simulink model "IEEE5BusSystemModel_opt_UFLS"  (R2019b)
settings: Solver=ode4  StartTime=0.0  StopTime=300  MaxStep=1e-4  RelTol=1e-3
InitFcn:
  | startup_RTS
values from neighbouring files (symbols this model uses):
  C = b/(2*pi*60*Zn)    [startup_RTS.m]
  C0 = C/3    [startup_RTS.m]
  dPLS1 = 0    [startup_RTS.m]
  dPLS2 = 0    [startup_RTS.m]
  dPLS3 = 0    [startup_RTS.m]
  dQLS1 = 0    [startup_RTS.m]
  dQLS2 = 0    [startup_RTS.m]
  dQLS3 = 0    [startup_RTS.m]
  fn = 50    [startup_RTS.m]
  In = Sn/(sqrt(3)*Vn)    [startup_RTS.m]
  L = x*Zn/(2*pi*60)    [startup_RTS.m]
  L0 = 3*L    [startup_RTS.m]
  len = ceil(0.95*300000*T_prop)    [startup_RTS.m]
  PL1 = 300e6    (= 300000000)    [startup_RTS.m]
  PL2 = 300e6    (= 300000000)    [startup_RTS.m]
  PL3 = 300e6    (= 300000000)    [startup_RTS.m]
  QL1 = 30e6    (= 30000000)    [startup_RTS.m]
  QL2 = 30e6    (= 30000000)    [startup_RTS.m]
  QL3 = 30e6    (= 30000000)    [startup_RTS.m]
  R = r*Zn    [startup_RTS.m]
  R0 = 3*R    [startup_RTS.m]
  Sn = 1000e6    (= 1000000000)    [startup_RTS.m]
  t_cont = 100    [startup_RTS.m]
  Vn = 345e3    (= 345000)    [startup_RTS.m]
undefined symbols (not defined in the file or in its folder): D1, Delta
libraries: powerlib x42, dspswit3 x10, powerlib_meascontrol x3, dspstat3 x3, sps_avr x3, spsExcitationSystemModel x3
(part 3 of 7)

== system IEEE5BusSystemModel_opt_UFLS/Subsystem1/PMU_e-IpDFT_P-class1/Ia_est ==
  signal : Inport
  Hit : Inport  Port=2
  dT [s] : Inport  Port=3
  dF [Hz] : Inport  Port=4
  Synchrophasor estimation : Subsystem
  mSDFT : Subsystem
  Frequency : Outport  VectorParamsAs1DForOutWhenUnconnected=off
  Amplitude : Outport  Port=2  VectorParamsAs1DForOutWhenUnconnected=off
  Phase : Outport  Port=3  VectorParamsAs1DForOutWhenUnconnected=off
  wires:
  dF [Hz]/1 -> Synchrophasor estimation/3(dF [Hz])
  Synchrophasor estimation/1(Frequency) -> Frequency/1
  signal/1 -> mSDFT/1(signal)
  mSDFT/1(DFT) -> Synchrophasor estimation/1(DFT)
  Synchrophasor estimation/2(Amplitude) -> Amplitude/1
  Synchrophasor estimation/3(Phase) -> Phase/1
  Hit/1 -> mSDFT/2(Hit)
  dT [s]/1 -> Synchrophasor estimation/2(dT [s])

== system IEEE5BusSystemModel_opt_UFLS/Subsystem2/PMU_e-IpDFT_P-class/Ia_est ==
  signal : Inport
  Hit : Inport  Port=2
  dT [s] : Inport  Port=3
  dF [Hz] : Inport  Port=4
  Synchrophasor estimation : Subsystem
  mSDFT : Subsystem
  Frequency : Outport  VectorParamsAs1DForOutWhenUnconnected=off
  Amplitude : Outport  Port=2  VectorParamsAs1DForOutWhenUnconnected=off
  Phase : Outport  Port=3  VectorParamsAs1DForOutWhenUnconnected=off
  wires:
  dF [Hz]/1 -> Synchrophasor estimation/3(dF [Hz])
  Synchrophasor estimation/1(Frequency) -> Frequency/1
  signal/1 -> mSDFT/1(signal)
  mSDFT/1(DFT) -> Synchrophasor estimation/1(DFT)
  Synchrophasor estimation/2(Amplitude) -> Amplitude/1
  Synchrophasor estimation/3(Phase) -> Phase/1
  Hit/1 -> mSDFT/2(Hit)
  dT [s]/1 -> Synchrophasor estimation/2(dT [s])

== system IEEE5BusSystemModel_opt_UFLS/Subsystem2/PMU_e-IpDFT_P-class1/Ia_est ==
  signal : Inport
  Hit : Inport  Port=2
  dT [s] : Inport  Port=3
  dF [Hz] : Inport  Port=4
  Synchrophasor estimation : Subsystem
  mSDFT : Subsystem
  Frequency : Outport  VectorParamsAs1DForOutWhenUnconnected=off
  Amplitude : Outport  Port=2  VectorParamsAs1DForOutWhenUnconnected=off
  Phase : Outport  Port=3  VectorParamsAs1DForOutWhenUnconnected=off
  wires:
  dT [s]/1 -> Synchrophasor estimation/2(dT [s])
  Hit/1 -> mSDFT/2(Hit)
  Synchrophasor estimation/3(Phase) -> Phase/1
  Synchrophasor estimation/2(Amplitude) -> Amplitude/1
  mSDFT/1(DFT) -> Synchrophasor estimation/1(DFT)
  signal/1 -> mSDFT/1(signal)
  Synchrophasor estimation/1(Frequency) -> Frequency/1
  dF [Hz]/1 -> Synchrophasor estimation/3(dF [Hz])

== system IEEE5BusSystemModel_opt_UFLS/Subsystem3/PMU_e-IpDFT_P-class/Ia_est ==
  signal : Inport
  Hit : Inport  Port=2
  dT [s] : Inport  Port=3
  dF [Hz] : Inport  Port=4
  Synchrophasor estimation : Subsystem
  mSDFT : Subsystem
  Frequency : Outport  VectorParamsAs1DForOutWhenUnconnected=off
  Amplitude : Outport  Port=2  VectorParamsAs1DForOutWhenUnconnected=off
  Phase : Outport  Port=3  VectorParamsAs1DForOutWhenUnconnected=off
  wires:
  dT [s]/1 -> Synchrophasor estimation/2(dT [s])
  Hit/1 -> mSDFT/2(Hit)
  Synchrophasor estimation/3(Phase) -> Phase/1
  Synchrophasor estimation/2(Amplitude) -> Amplitude/1
  mSDFT/1(DFT) -> Synchrophasor estimation/1(DFT)
  signal/1 -> mSDFT/1(signal)
  Synchrophasor estimation/1(Frequency) -> Frequency/1
  dF [Hz]/1 -> Synchrophasor estimation/3(dF [Hz])

== system IEEE5BusSystemModel_opt_UFLS/Subsystem3/PMU_e-IpDFT_P-class1/Ia_est ==
  signal : Inport
  Hit : Inport  Port=2
  dT [s] : Inport  Port=3
  dF [Hz] : Inport  Port=4
  Synchrophasor estimation : Subsystem
  mSDFT : Subsystem
  Frequency : Outport  VectorParamsAs1DForOutWhenUnconnected=off
  Amplitude : Outport  Port=2  VectorParamsAs1DForOutWhenUnconnected=off
  Phase : Outport  Port=3  VectorParamsAs1DForOutWhenUnconnected=off
  wires:
  dF [Hz]/1 -> Synchrophasor estimation/3(dF [Hz])
  Synchrophasor estimation/1(Frequency) -> Frequency/1
  signal/1 -> mSDFT/1(signal)
  mSDFT/1(DFT) -> Synchrophasor estimation/1(DFT)
  Synchrophasor estimation/2(Amplitude) -> Amplitude/1
  Synchrophasor estimation/3(Phase) -> Phase/1
  Hit/1 -> mSDFT/2(Hit)
  dT [s]/1 -> Synchrophasor estimation/2(dT [s])

== system IEEE5BusSystemModel_opt_UFLS/Subsystem4/PMU_e-IpDFT_P-class/Ia_est ==
  signal : Inport
  Hit : Inport  Port=2
  dT [s] : Inport  Port=3
  dF [Hz] : Inport  Port=4
  Synchrophasor estimation : Subsystem
  mSDFT : Subsystem
  Frequency : Outport  VectorParamsAs1DForOutWhenUnconnected=off
  Amplitude : Outport  Port=2  VectorParamsAs1DForOutWhenUnconnected=off
  Phase : Outport  Port=3  VectorParamsAs1DForOutWhenUnconnected=off
  wires:
  dF [Hz]/1 -> Synchrophasor estimation/3(dF [Hz])
  Synchrophasor estimation/1(Frequency) -> Frequency/1
  signal/1 -> mSDFT/1(signal)
  mSDFT/1(DFT) -> Synchrophasor estimation/1(DFT)
  Synchrophasor estimation/2(Amplitude) -> Amplitude/1
  Synchrophasor estimation/3(Phase) -> Phase/1
  Hit/1 -> mSDFT/2(Hit)
  dT [s]/1 -> Synchrophasor estimation/2(dT [s])

== system IEEE5BusSystemModel_opt_UFLS/Subsystem4/PMU_e-IpDFT_P-class1/Ia_est ==
  signal : Inport
  Hit : Inport  Port=2
  dT [s] : Inport  Port=3
  dF [Hz] : Inport  Port=4
  Synchrophasor estimation : Subsystem
  mSDFT : Subsystem
  Frequency : Outport  VectorParamsAs1DForOutWhenUnconnected=off
  Amplitude : Outport  Port=2  VectorParamsAs1DForOutWhenUnconnected=off
  Phase : Outport  Port=3  VectorParamsAs1DForOutWhenUnconnected=off
  wires:
  dT [s]/1 -> Synchrophasor estimation/2(dT [s])
  Hit/1 -> mSDFT/2(Hit)
  Synchrophasor estimation/3(Phase) -> Phase/1
  Synchrophasor estimation/2(Amplitude) -> Amplitude/1
  mSDFT/1(DFT) -> Synchrophasor estimation/1(DFT)
  signal/1 -> mSDFT/1(signal)
  Synchrophasor estimation/1(Frequency) -> Frequency/1
  dF [Hz]/1 -> Synchrophasor estimation/3(dF [Hz])

== system IEEE5BusSystemModel_opt_UFLS/Subsystem5/PMU_e-IpDFT_P-class/Ia_est ==
  signal : Inport
  Hit : Inport  Port=2
  dT [s] : Inport  Port=3
  dF [Hz] : Inport  Port=4
  Synchrophasor estimation : Subsystem
  mSDFT : Subsystem
  Frequency : Outport  VectorParamsAs1DForOutWhenUnconnected=off
  Amplitude : Outport  Port=2  VectorParamsAs1DForOutWhenUnconnected=off
  Phase : Outport  Port=3  VectorParamsAs1DForOutWhenUnconnected=off
  wires:
  dF [Hz]/1 -> Synchrophasor estimation/3(dF [Hz])
  Synchrophasor estimation/1(Frequency) -> Frequency/1
  signal/1 -> mSDFT/1(signal)
  mSDFT/1(DFT) -> Synchrophasor estimation/1(DFT)
  Synchrophasor estimation/2(Amplitude) -> Amplitude/1
  Synchrophasor estimation/3(Phase) -> Phase/1
  Hit/1 -> mSDFT/2(Hit)
  dT [s]/1 -> Synchrophasor estimation/2(dT [s])

== system IEEE5BusSystemModel_opt_UFLS/Subsystem5/PMU_e-IpDFT_P-class1/Ia_est ==
  signal : Inport
  Hit : Inport  Port=2
  dT [s] : Inport  Port=3
  dF [Hz] : Inport  Port=4
  Synchrophasor estimation : Subsystem
  mSDFT : Subsystem
  Frequency : Outport  VectorParamsAs1DForOutWhenUnconnected=off
  Amplitude : Outport  Port=2  VectorParamsAs1DForOutWhenUnconnected=off
  Phase : Outport  Port=3  VectorParamsAs1DForOutWhenUnconnected=off
  wires:
  dT [s]/1 -> Synchrophasor estimation/2(dT [s])
  Hit/1 -> mSDFT/2(Hit)
  Synchrophasor estimation/3(Phase) -> Phase/1
  Synchrophasor estimation/2(Amplitude) -> Amplitude/1
  mSDFT/1(DFT) -> Synchrophasor estimation/1(DFT)
  signal/1 -> mSDFT/1(signal)
  Synchrophasor estimation/1(Frequency) -> Frequency/1
  dF [Hz]/1 -> Synchrophasor estimation/3(dF [Hz])

== system IEEE5BusSystemModel_opt_UFLS/Subsystem1/PMU_e-IpDFT_P-class/Ia_est/Synchrophasor estimation ==
  DFT : Inport
  dT [s] : Inport  Port=2
  dF [Hz] : Inport  Port=3
  Amplitude - 1 : Subsystem
  Amplitude - 2 : Subsystem
  Complex to Magnitude-Angle1 : ComplexToMagnitudeAngle
  Complex to Magnitude-Angle2 : ComplexToMagnitudeAngle
  Demux1 : Demux  Outputs=5
  Frequency - 2 : Subsystem
  Hanning(Kmax) : Subsystem
  Hanning(Kmax+1) : Subsystem
  Hanning(Kmax-1) : Subsystem
  Phase - 2 : Subsystem
  Terminator : Terminator
  Terminator1 : Terminator
  "delta - 1 " : Subsystem
  delta - 2 : Subsystem
  epsilon : Subsystem
  spectral leakage compensation : Subsystem
  Frequency : Outport  VectorParamsAs1DForOutWhenUnconnected=off
  Amplitude : Outport  Port=2  VectorParamsAs1DForOutWhenUnconnected=off
  Phase : Outport  Port=3  VectorParamsAs1DForOutWhenUnconnected=off
  wires:
  DFT/1 -> Demux1/1
  Frequency - 2/1(frequency) -> Phase - 2/3(freq), Frequency/1
  Amplitude - 2/1(amplitude) -> Amplitude/1
  Demux1/5 -> Hanning(Kmax+1)/3(Kmax+2)
  Demux1/1 -> Hanning(Kmax-1)/1(Kmax-2)
  Demux1/2 -> Hanning(Kmax)/1(Kmax-1), Hanning(Kmax-1)/2(Kmax-1)
  Demux1/3 -> Hanning(Kmax-1)/3(Kmax), Hanning(Kmax+1)/1(Kmax), Hanning(Kmax)/2(Kmax)
  Demux1/4 -> Hanning(Kmax+1)/2(Kmax+1), Hanning(Kmax)/3(Kmax+1)
  Hanning(Kmax+1)/1(Hanning out) -> epsilon/2(X (k max+1))
  Hanning(Kmax)/1(Hanning out) -> "delta - 1 "/1(X (k max)), Amplitude - 1/2((X k_max)), spectral leakage compensation/4(X (k max))
  epsilon/1(X (Kmax + epsilon)) -> "delta - 1 "/2(X (k max + epsilon)), spectral leakage compensation/3(X (k max + epsilon))
  epsilon/2(epsilon) -> spectral leakage compensation/5(epsilon), delta - 2/3(epsilon), "delta - 1 "/3(epsilon)
  "delta - 1 "/1(delta) -> spectral leakage compensation/2(delta), Amplitude - 1/1(delta)
  spectral leakage compensation/1(X(k max)) -> delta - 2/1(X (k max)), Complex to Magnitude-Angle2/1, Amplitude - 2/2((X k_max))
  spectral leakage compensation/2(X(k max+epsilon)) -> delta - 2/2(X (k max + epsilon))
  delta - 2/1(delta) -> Frequency - 2/1(delta), Phase - 2/2(delta), Amplitude - 2/1(delta)
  Phase - 2/1(phase) -> Phase/1
  Complex to Magnitude-Angle1/2 -> spectral leakage compensation/6(ph X(k-1))
  Complex to Magnitude-Angle1/1 -> Terminator/1
  Complex to Magnitude-Angle2/2 -> Phase - 2/1(X k_max phase)
  Complex to Magnitude-Angle2/1 -> Terminator1/1
  dT [s]/1 -> Phase - 2/4(dT [s])
  Amplitude - 1/1(amplitude) -> spectral leakage compensation/1(Amplitude)
  Hanning(Kmax-1)/1(Hanning out) -> Complex to Magnitude-Angle1/1, epsilon/1(X (k max -1))
  dF [Hz]/1 -> Frequency - 2/2(dF [Hz])

== system IEEE5BusSystemModel_opt_UFLS/Subsystem1/PMU_e-IpDFT_P-class/Ia_est/mSDFT ==
  signal : Inport
  Hit : Inport  Port=2
  Delay_M : Delay  DelayLength=M  SampleTime=Ts_p
  Kmax : Subsystem
  Kmax+1 : Subsystem
  Kmax+2 : Subsystem
  Kmax-1 : Subsystem
  Kmax-2 : Subsystem
  Mux : Mux  Inputs=5
  DFT : Outport  VectorParamsAs1DForOutWhenUnconnected=off
  wires:
  Mux/1 -> DFT/1
  Kmax+2/1(X(k)) -> Mux/5
  Kmax+1/1(X(k)) -> Mux/4
  Kmax/1(X(k)) -> Mux/3
  Kmax-1/1(X(k)) -> Mux/2
  Kmax-2/1(X(k)) -> Mux/1
  signal/1 -> Kmax-2/1(x(n)), Kmax-1/1(x(n)), Kmax+2/1(x(n)), Kmax+1/1(x(n)), Kmax/1(x(n)), Delay_M/1
  Delay_M/1 -> Kmax/2(x(n-M)), Kmax+1/2(x(n-M)), Kmax+2/2(x(n-M)), Kmax-1/2(x(n-M)), Kmax-2/2(x(n-M))
  Hit/1 -> Kmax-2/3(trigger), Kmax-1/3(trigger), Kmax/3(trigger), Kmax+1/3(trigger), Kmax+2/3(trigger)

== system IEEE5BusSystemModel_opt_UFLS/Subsystem1/PMU_e-IpDFT_P-class1/Ia_est/Synchrophasor estimation ==
  DFT : Inport
  dT [s] : Inport  Port=2
  dF [Hz] : Inport  Port=3
  Amplitude - 1 : Subsystem
  Amplitude - 2 : Subsystem
  Complex to Magnitude-Angle1 : ComplexToMagnitudeAngle
  Complex to Magnitude-Angle2 : ComplexToMagnitudeAngle
  Demux1 : Demux  Outputs=5
  Frequency - 2 : Subsystem
  Hanning(Kmax) : Subsystem
  Hanning(Kmax+1) : Subsystem
  Hanning(Kmax-1) : Subsystem
  Phase - 2 : Subsystem
  Terminator : Terminator
  Terminator1 : Terminator
  "delta - 1 " : Subsystem
  delta - 2 : Subsystem
  epsilon : Subsystem
  spectral leakage compensation : Subsystem
  Frequency : Outport  VectorParamsAs1DForOutWhenUnconnected=off
  Amplitude : Outport  Port=2  VectorParamsAs1DForOutWhenUnconnected=off
  Phase : Outport  Port=3  VectorParamsAs1DForOutWhenUnconnected=off
  wires:
  dF [Hz]/1 -> Frequency - 2/2(dF [Hz])
  Hanning(Kmax-1)/1(Hanning out) -> epsilon/1(X (k max -1)), Complex to Magnitude-Angle1/1
  Amplitude - 1/1(amplitude) -> spectral leakage compensation/1(Amplitude)
  dT [s]/1 -> Phase - 2/4(dT [s])
  Complex to Magnitude-Angle2/1 -> Terminator1/1
  Complex to Magnitude-Angle2/2 -> Phase - 2/1(X k_max phase)
  Complex to Magnitude-Angle1/1 -> Terminator/1
  Complex to Magnitude-Angle1/2 -> spectral leakage compensation/6(ph X(k-1))
  Phase - 2/1(phase) -> Phase/1
  delta - 2/1(delta) -> Amplitude - 2/1(delta), Phase - 2/2(delta), Frequency - 2/1(delta)
  spectral leakage compensation/2(X(k max+epsilon)) -> delta - 2/2(X (k max + epsilon))
  spectral leakage compensation/1(X(k max)) -> Amplitude - 2/2((X k_max)), Complex to Magnitude-Angle2/1, delta - 2/1(X (k max))
  "delta - 1 "/1(delta) -> Amplitude - 1/1(delta), spectral leakage compensation/2(delta)
  epsilon/2(epsilon) -> "delta - 1 "/3(epsilon), delta - 2/3(epsilon), spectral leakage compensation/5(epsilon)
  epsilon/1(X (Kmax + epsilon)) -> spectral leakage compensation/3(X (k max + epsilon)), "delta - 1 "/2(X (k max + epsilon))
  Hanning(Kmax)/1(Hanning out) -> spectral leakage compensation/4(X (k max)), Amplitude - 1/2((X k_max)), "delta - 1 "/1(X (k max))
  Hanning(Kmax+1)/1(Hanning out) -> epsilon/2(X (k max+1))
  Demux1/4 -> Hanning(Kmax)/3(Kmax+1), Hanning(Kmax+1)/2(Kmax+1)
  Demux1/3 -> Hanning(Kmax)/2(Kmax), Hanning(Kmax+1)/1(Kmax), Hanning(Kmax-1)/3(Kmax)
  Demux1/2 -> Hanning(Kmax-1)/2(Kmax-1), Hanning(Kmax)/1(Kmax-1)
  Demux1/1 -> Hanning(Kmax-1)/1(Kmax-2)
  Demux1/5 -> Hanning(Kmax+1)/3(Kmax+2)
  Amplitude - 2/1(amplitude) -> Amplitude/1
  Frequency - 2/1(frequency) -> Frequency/1, Phase - 2/3(freq)
  DFT/1 -> Demux1/1

== system IEEE5BusSystemModel_opt_UFLS/Subsystem1/PMU_e-IpDFT_P-class1/Ia_est/mSDFT ==
  signal : Inport
  Hit : Inport  Port=2
  Delay_M : Delay  DelayLength=M  SampleTime=Ts_p
  Kmax : Subsystem
  Kmax+1 : Subsystem
  Kmax+2 : Subsystem
  Kmax-1 : Subsystem
  Kmax-2 : Subsystem
  Mux : Mux  Inputs=5
  DFT : Outport  VectorParamsAs1DForOutWhenUnconnected=off
  wires:
  Hit/1 -> Kmax+2/3(trigger), Kmax+1/3(trigger), Kmax/3(trigger), Kmax-1/3(trigger), Kmax-2/3(trigger)
  Delay_M/1 -> Kmax-2/2(x(n-M)), Kmax-1/2(x(n-M)), Kmax+2/2(x(n-M)), Kmax+1/2(x(n-M)), Kmax/2(x(n-M))
  signal/1 -> Delay_M/1, Kmax/1(x(n)), Kmax+1/1(x(n)), Kmax+2/1(x(n)), Kmax-1/1(x(n)), Kmax-2/1(x(n))
  Kmax-2/1(X(k)) -> Mux/1
  Kmax-1/1(X(k)) -> Mux/2
  Kmax/1(X(k)) -> Mux/3
  Kmax+1/1(X(k)) -> Mux/4
  Kmax+2/1(X(k)) -> Mux/5
  Mux/1 -> DFT/1

== system IEEE5BusSystemModel_opt_UFLS/Subsystem2/PMU_e-IpDFT_P-class/Ia_est/Synchrophasor estimation ==
  DFT : Inport
  dT [s] : Inport  Port=2
  dF [Hz] : Inport  Port=3
  Amplitude - 1 : Subsystem
  Amplitude - 2 : Subsystem
  Complex to Magnitude-Angle1 : ComplexToMagnitudeAngle
  Complex to Magnitude-Angle2 : ComplexToMagnitudeAngle
  Demux1 : Demux  Outputs=5
  Frequency - 2 : Subsystem
  Hanning(Kmax) : Subsystem
  Hanning(Kmax+1) : Subsystem
  Hanning(Kmax-1) : Subsystem
  Phase - 2 : Subsystem
  Terminator : Terminator
  Terminator1 : Terminator
  "delta - 1 " : Subsystem
  delta - 2 : Subsystem
  epsilon : Subsystem
  spectral leakage compensation : Subsystem
  Frequency : Outport  VectorParamsAs1DForOutWhenUnconnected=off
  Amplitude : Outport  Port=2  VectorParamsAs1DForOutWhenUnconnected=off
  Phase : Outport  Port=3  VectorParamsAs1DForOutWhenUnconnected=off
  wires:
  dF [Hz]/1 -> Frequency - 2/2(dF [Hz])
  Hanning(Kmax-1)/1(Hanning out) -> epsilon/1(X (k max -1)), Complex to Magnitude-Angle1/1
  Amplitude - 1/1(amplitude) -> spectral leakage compensation/1(Amplitude)
  dT [s]/1 -> Phase - 2/4(dT [s])
  Complex to Magnitude-Angle2/1 -> Terminator1/1
  Complex to Magnitude-Angle2/2 -> Phase - 2/1(X k_max phase)
  Complex to Magnitude-Angle1/1 -> Terminator/1
  Complex to Magnitude-Angle1/2 -> spectral leakage compensation/6(ph X(k-1))
  Phase - 2/1(phase) -> Phase/1
  delta - 2/1(delta) -> Amplitude - 2/1(delta), Phase - 2/2(delta), Frequency - 2/1(delta)
  spectral leakage compensation/2(X(k max+epsilon)) -> delta - 2/2(X (k max + epsilon))
  spectral leakage compensation/1(X(k max)) -> Amplitude - 2/2((X k_max)), Complex to Magnitude-Angle2/1, delta - 2/1(X (k max))
  "delta - 1 "/1(delta) -> Amplitude - 1/1(delta), spectral leakage compensation/2(delta)
  epsilon/2(epsilon) -> "delta - 1 "/3(epsilon), delta - 2/3(epsilon), spectral leakage compensation/5(epsilon)
  epsilon/1(X (Kmax + epsilon)) -> spectral leakage compensation/3(X (k max + epsilon)), "delta - 1 "/2(X (k max + epsilon))
  Hanning(Kmax)/1(Hanning out) -> spectral leakage compensation/4(X (k max)), Amplitude - 1/2((X k_max)), "delta - 1 "/1(X (k max))
  Hanning(Kmax+1)/1(Hanning out) -> epsilon/2(X (k max+1))
  Demux1/4 -> Hanning(Kmax)/3(Kmax+1), Hanning(Kmax+1)/2(Kmax+1)
  Demux1/3 -> Hanning(Kmax)/2(Kmax), Hanning(Kmax+1)/1(Kmax), Hanning(Kmax-1)/3(Kmax)
  Demux1/2 -> Hanning(Kmax-1)/2(Kmax-1), Hanning(Kmax)/1(Kmax-1)
  Demux1/1 -> Hanning(Kmax-1)/1(Kmax-2)
  Demux1/5 -> Hanning(Kmax+1)/3(Kmax+2)
  Amplitude - 2/1(amplitude) -> Amplitude/1
  Frequency - 2/1(frequency) -> Frequency/1, Phase - 2/3(freq)
  DFT/1 -> Demux1/1

== system IEEE5BusSystemModel_opt_UFLS/Subsystem2/PMU_e-IpDFT_P-class/Ia_est/mSDFT ==
  signal : Inport
  Hit : Inport  Port=2
  Delay_M : Delay  DelayLength=M  SampleTime=Ts_p
  Kmax : Subsystem
  Kmax+1 : Subsystem
  Kmax+2 : Subsystem
  Kmax-1 : Subsystem
  Kmax-2 : Subsystem
  Mux : Mux  Inputs=5
  DFT : Outport  VectorParamsAs1DForOutWhenUnconnected=off
  wires:
  Hit/1 -> Kmax+2/3(trigger), Kmax+1/3(trigger), Kmax/3(trigger), Kmax-1/3(trigger), Kmax-2/3(trigger)
  Delay_M/1 -> Kmax-2/2(x(n-M)), Kmax-1/2(x(n-M)), Kmax+2/2(x(n-M)), Kmax+1/2(x(n-M)), Kmax/2(x(n-M))
  signal/1 -> Delay_M/1, Kmax/1(x(n)), Kmax+1/1(x(n)), Kmax+2/1(x(n)), Kmax-1/1(x(n)), Kmax-2/1(x(n))
  Kmax-2/1(X(k)) -> Mux/1
  Kmax-1/1(X(k)) -> Mux/2
  Kmax/1(X(k)) -> Mux/3
  Kmax+1/1(X(k)) -> Mux/4
  Kmax+2/1(X(k)) -> Mux/5
  Mux/1 -> DFT/1

== system IEEE5BusSystemModel_opt_UFLS/Subsystem2/PMU_e-IpDFT_P-class1/Ia_est/Synchrophasor estimation ==
  DFT : Inport
  dT [s] : Inport  Port=2
  dF [Hz] : Inport  Port=3
  Amplitude - 1 : Subsystem
  Amplitude - 2 : Subsystem
  Complex to Magnitude-Angle1 : ComplexToMagnitudeAngle
  Complex to Magnitude-Angle2 : ComplexToMagnitudeAngle
  Demux1 : Demux  Outputs=5
  Frequency - 2 : Subsystem
  Hanning(Kmax) : Subsystem
  Hanning(Kmax+1) : Subsystem
  Hanning(Kmax-1) : Subsystem
  Phase - 2 : Subsystem
  Terminator : Terminator
  Terminator1 : Terminator
  "delta - 1 " : Subsystem
  delta - 2 : Subsystem
  epsilon : Subsystem
  spectral leakage compensation : Subsystem
  Frequency : Outport  VectorParamsAs1DForOutWhenUnconnected=off
  Amplitude : Outport  Port=2  VectorParamsAs1DForOutWhenUnconnected=off
  Phase : Outport  Port=3  VectorParamsAs1DForOutWhenUnconnected=off
  wires:
  DFT/1 -> Demux1/1
  Frequency - 2/1(frequency) -> Phase - 2/3(freq), Frequency/1
  Amplitude - 2/1(amplitude) -> Amplitude/1
  Demux1/5 -> Hanning(Kmax+1)/3(Kmax+2)
  Demux1/1 -> Hanning(Kmax-1)/1(Kmax-2)
  Demux1/2 -> Hanning(Kmax)/1(Kmax-1), Hanning(Kmax-1)/2(Kmax-1)
  Demux1/3 -> Hanning(Kmax-1)/3(Kmax), Hanning(Kmax+1)/1(Kmax), Hanning(Kmax)/2(Kmax)
  Demux1/4 -> Hanning(Kmax+1)/2(Kmax+1), Hanning(Kmax)/3(Kmax+1)
  Hanning(Kmax+1)/1(Hanning out) -> epsilon/2(X (k max+1))
  Hanning(Kmax)/1(Hanning out) -> "delta - 1 "/1(X (k max)), Amplitude - 1/2((X k_max)), spectral leakage compensation/4(X (k max))
  epsilon/1(X (Kmax + epsilon)) -> "delta - 1 "/2(X (k max + epsilon)), spectral leakage compensation/3(X (k max + epsilon))
  epsilon/2(epsilon) -> spectral leakage compensation/5(epsilon), delta - 2/3(epsilon), "delta - 1 "/3(epsilon)
  "delta - 1 "/1(delta) -> spectral leakage compensation/2(delta), Amplitude - 1/1(delta)
  spectral leakage compensation/1(X(k max)) -> delta - 2/1(X (k max)), Complex to Magnitude-Angle2/1, Amplitude - 2/2((X k_max))
  spectral leakage compensation/2(X(k max+epsilon)) -> delta - 2/2(X (k max + epsilon))
  delta - 2/1(delta) -> Frequency - 2/1(delta), Phase - 2/2(delta), Amplitude - 2/1(delta)
  Phase - 2/1(phase) -> Phase/1
  Complex to Magnitude-Angle1/2 -> spectral leakage compensation/6(ph X(k-1))
  Complex to Magnitude-Angle1/1 -> Terminator/1
  Complex to Magnitude-Angle2/2 -> Phase - 2/1(X k_max phase)
  Complex to Magnitude-Angle2/1 -> Terminator1/1
  dT [s]/1 -> Phase - 2/4(dT [s])
  Amplitude - 1/1(amplitude) -> spectral leakage compensation/1(Amplitude)
  Hanning(Kmax-1)/1(Hanning out) -> Complex to Magnitude-Angle1/1, epsilon/1(X (k max -1))
  dF [Hz]/1 -> Frequency - 2/2(dF [Hz])

== system IEEE5BusSystemModel_opt_UFLS/Subsystem2/PMU_e-IpDFT_P-class1/Ia_est/mSDFT ==
  signal : Inport
  Hit : Inport  Port=2
  Delay_M : Delay  DelayLength=M  SampleTime=Ts_p
  Kmax : Subsystem
  Kmax+1 : Subsystem
  Kmax+2 : Subsystem
  Kmax-1 : Subsystem
  Kmax-2 : Subsystem
  Mux : Mux  Inputs=5
  DFT : Outport  VectorParamsAs1DForOutWhenUnconnected=off
  wires:
  Mux/1 -> DFT/1
  Kmax+2/1(X(k)) -> Mux/5
  Kmax+1/1(X(k)) -> Mux/4
  Kmax/1(X(k)) -> Mux/3
  Kmax-1/1(X(k)) -> Mux/2
  Kmax-2/1(X(k)) -> Mux/1
  signal/1 -> Kmax-2/1(x(n)), Kmax-1/1(x(n)), Kmax+2/1(x(n)), Kmax+1/1(x(n)), Kmax/1(x(n)), Delay_M/1
  Delay_M/1 -> Kmax/2(x(n-M)), Kmax+1/2(x(n-M)), Kmax+2/2(x(n-M)), Kmax-1/2(x(n-M)), Kmax-2/2(x(n-M))
  Hit/1 -> Kmax-2/3(trigger), Kmax-1/3(trigger), Kmax/3(trigger), Kmax+1/3(trigger), Kmax+2/3(trigger)

== system IEEE5BusSystemModel_opt_UFLS/Subsystem3/PMU_e-IpDFT_P-class/Ia_est/Synchrophasor estimation ==
  DFT : Inport
  dT [s] : Inport  Port=2
  dF [Hz] : Inport  Port=3
  Amplitude - 1 : Subsystem
  Amplitude - 2 : Subsystem
  Complex to Magnitude-Angle1 : ComplexToMagnitudeAngle
  Complex to Magnitude-Angle2 : ComplexToMagnitudeAngle
  Demux1 : Demux  Outputs=5
  Frequency - 2 : Subsystem
  Hanning(Kmax) : Subsystem
  Hanning(Kmax+1) : Subsystem
  Hanning(Kmax-1) : Subsystem
  Phase - 2 : Subsystem
  Terminator : Terminator
  Terminator1 : Terminator
  "delta - 1 " : Subsystem
  delta - 2 : Subsystem
  epsilon : Subsystem
  spectral leakage compensation : Subsystem
  Frequency : Outport  VectorParamsAs1DForOutWhenUnconnected=off
  Amplitude : Outport  Port=2  VectorParamsAs1DForOutWhenUnconnected=off
  Phase : Outport  Port=3  VectorParamsAs1DForOutWhenUnconnected=off
  wires:
  DFT/1 -> Demux1/1
  Frequency - 2/1(frequency) -> Phase - 2/3(freq), Frequency/1
  Amplitude - 2/1(amplitude) -> Amplitude/1
  Demux1/5 -> Hanning(Kmax+1)/3(Kmax+2)
  Demux1/1 -> Hanning(Kmax-1)/1(Kmax-2)
  Demux1/2 -> Hanning(Kmax)/1(Kmax-1), Hanning(Kmax-1)/2(Kmax-1)
  Demux1/3 -> Hanning(Kmax-1)/3(Kmax), Hanning(Kmax+1)/1(Kmax), Hanning(Kmax)/2(Kmax)
  Demux1/4 -> Hanning(Kmax+1)/2(Kmax+1), Hanning(Kmax)/3(Kmax+1)
  Hanning(Kmax+1)/1(Hanning out) -> epsilon/2(X (k max+1))
  Hanning(Kmax)/1(Hanning out) -> "delta - 1 "/1(X (k max)), Amplitude - 1/2((X k_max)), spectral leakage compensation/4(X (k max))
  epsilon/1(X (Kmax + epsilon)) -> "delta - 1 "/2(X (k max + epsilon)), spectral leakage compensation/3(X (k max + epsilon))
  epsilon/2(epsilon) -> spectral leakage compensation/5(epsilon), delta - 2/3(epsilon), "delta - 1 "/3(epsilon)
  "delta - 1 "/1(delta) -> spectral leakage compensation/2(delta), Amplitude - 1/1(delta)
  spectral leakage compensation/1(X(k max)) -> delta - 2/1(X (k max)), Complex to Magnitude-Angle2/1, Amplitude - 2/2((X k_max))
  spectral leakage compensation/2(X(k max+epsilon)) -> delta - 2/2(X (k max + epsilon))
  delta - 2/1(delta) -> Frequency - 2/1(delta), Phase - 2/2(delta), Amplitude - 2/1(delta)
  Phase - 2/1(phase) -> Phase/1
  Complex to Magnitude-Angle1/2 -> spectral leakage compensation/6(ph X(k-1))
  Complex to Magnitude-Angle1/1 -> Terminator/1
  Complex to Magnitude-Angle2/2 -> Phase - 2/1(X k_max phase)
  Complex to Magnitude-Angle2/1 -> Terminator1/1
  dT [s]/1 -> Phase - 2/4(dT [s])
  Amplitude - 1/1(amplitude) -> spectral leakage compensation/1(Amplitude)
  Hanning(Kmax-1)/1(Hanning out) -> Complex to Magnitude-Angle1/1, epsilon/1(X (k max -1))
  dF [Hz]/1 -> Frequency - 2/2(dF [Hz])

== system IEEE5BusSystemModel_opt_UFLS/Subsystem3/PMU_e-IpDFT_P-class/Ia_est/mSDFT ==
  signal : Inport
  Hit : Inport  Port=2
  Delay_M : Delay  DelayLength=M  SampleTime=Ts_p
  Kmax : Subsystem
  Kmax+1 : Subsystem
  Kmax+2 : Subsystem
  Kmax-1 : Subsystem
  Kmax-2 : Subsystem
  Mux : Mux  Inputs=5
  DFT : Outport  VectorParamsAs1DForOutWhenUnconnected=off
  wires:
  Mux/1 -> DFT/1
  Kmax+2/1(X(k)) -> Mux/5
  Kmax+1/1(X(k)) -> Mux/4
  Kmax/1(X(k)) -> Mux/3
  Kmax-1/1(X(k)) -> Mux/2
  Kmax-2/1(X(k)) -> Mux/1
  signal/1 -> Kmax-2/1(x(n)), Kmax-1/1(x(n)), Kmax+2/1(x(n)), Kmax+1/1(x(n)), Kmax/1(x(n)), Delay_M/1
  Delay_M/1 -> Kmax/2(x(n-M)), Kmax+1/2(x(n-M)), Kmax+2/2(x(n-M)), Kmax-1/2(x(n-M)), Kmax-2/2(x(n-M))
  Hit/1 -> Kmax-2/3(trigger), Kmax-1/3(trigger), Kmax/3(trigger), Kmax+1/3(trigger), Kmax+2/3(trigger)

== system IEEE5BusSystemModel_opt_UFLS/Subsystem3/PMU_e-IpDFT_P-class1/Ia_est/Synchrophasor estimation ==
  DFT : Inport
  dT [s] : Inport  Port=2
  dF [Hz] : Inport  Port=3
  Amplitude - 1 : Subsystem
  Amplitude - 2 : Subsystem
  Complex to Magnitude-Angle1 : ComplexToMagnitudeAngle
  Complex to Magnitude-Angle2 : ComplexToMagnitudeAngle
  Demux1 : Demux  Outputs=5
  Frequency - 2 : Subsystem
  Hanning(Kmax) : Subsystem
  Hanning(Kmax+1) : Subsystem
  Hanning(Kmax-1) : Subsystem
  Phase - 2 : Subsystem
  Terminator : Terminator
  Terminator1 : Terminator
  "delta - 1 " : Subsystem
  delta - 2 : Subsystem
  epsilon : Subsystem
  spectral leakage compensation : Subsystem
  Frequency : Outport  VectorParamsAs1DForOutWhenUnconnected=off
  Amplitude : Outport  Port=2  VectorParamsAs1DForOutWhenUnconnected=off
  Phase : Outport  Port=3  VectorParamsAs1DForOutWhenUnconnected=off
  wires:
  dF [Hz]/1 -> Frequency - 2/2(dF [Hz])
  Hanning(Kmax-1)/1(Hanning out) -> epsilon/1(X (k max -1)), Complex to Magnitude-Angle1/1
  Amplitude - 1/1(amplitude) -> spectral leakage compensation/1(Amplitude)
  dT [s]/1 -> Phase - 2/4(dT [s])
  Complex to Magnitude-Angle2/1 -> Terminator1/1
  Complex to Magnitude-Angle2/2 -> Phase - 2/1(X k_max phase)
  Complex to Magnitude-Angle1/1 -> Terminator/1
  Complex to Magnitude-Angle1/2 -> spectral leakage compensation/6(ph X(k-1))
  Phase - 2/1(phase) -> Phase/1
  delta - 2/1(delta) -> Amplitude - 2/1(delta), Phase - 2/2(delta), Frequency - 2/1(delta)
  spectral leakage compensation/2(X(k max+epsilon)) -> delta - 2/2(X (k max + epsilon))
  spectral leakage compensation/1(X(k max)) -> Amplitude - 2/2((X k_max)), Complex to Magnitude-Angle2/1, delta - 2/1(X (k max))
  "delta - 1 "/1(delta) -> Amplitude - 1/1(delta), spectral leakage compensation/2(delta)
  epsilon/2(epsilon) -> "delta - 1 "/3(epsilon), delta - 2/3(epsilon), spectral leakage compensation/5(epsilon)
  epsilon/1(X (Kmax + epsilon)) -> spectral leakage compensation/3(X (k max + epsilon)), "delta - 1 "/2(X (k max + epsilon))
  Hanning(Kmax)/1(Hanning out) -> spectral leakage compensation/4(X (k max)), Amplitude - 1/2((X k_max)), "delta - 1 "/1(X (k max))
  Hanning(Kmax+1)/1(Hanning out) -> epsilon/2(X (k max+1))
  Demux1/4 -> Hanning(Kmax)/3(Kmax+1), Hanning(Kmax+1)/2(Kmax+1)
  Demux1/3 -> Hanning(Kmax)/2(Kmax), Hanning(Kmax+1)/1(Kmax), Hanning(Kmax-1)/3(Kmax)
  Demux1/2 -> Hanning(Kmax-1)/2(Kmax-1), Hanning(Kmax)/1(Kmax-1)
  Demux1/1 -> Hanning(Kmax-1)/1(Kmax-2)
  Demux1/5 -> Hanning(Kmax+1)/3(Kmax+2)
  Amplitude - 2/1(amplitude) -> Amplitude/1
  Frequency - 2/1(frequency) -> Frequency/1, Phase - 2/3(freq)
  DFT/1 -> Demux1/1

== system IEEE5BusSystemModel_opt_UFLS/Subsystem3/PMU_e-IpDFT_P-class1/Ia_est/mSDFT ==
  signal : Inport
  Hit : Inport  Port=2
  Delay_M : Delay  DelayLength=M  SampleTime=Ts_p
  Kmax : Subsystem
  Kmax+1 : Subsystem
  Kmax+2 : Subsystem
  Kmax-1 : Subsystem
  Kmax-2 : Subsystem
  Mux : Mux  Inputs=5
  DFT : Outport  VectorParamsAs1DForOutWhenUnconnected=off
  wires:
  Hit/1 -> Kmax+2/3(trigger), Kmax+1/3(trigger), Kmax/3(trigger), Kmax-1/3(trigger), Kmax-2/3(trigger)
  Delay_M/1 -> Kmax-2/2(x(n-M)), Kmax-1/2(x(n-M)), Kmax+2/2(x(n-M)), Kmax+1/2(x(n-M)), Kmax/2(x(n-M))
  signal/1 -> Delay_M/1, Kmax/1(x(n)), Kmax+1/1(x(n)), Kmax+2/1(x(n)), Kmax-1/1(x(n)), Kmax-2/1(x(n))
  Kmax-2/1(X(k)) -> Mux/1
  Kmax-1/1(X(k)) -> Mux/2
  Kmax/1(X(k)) -> Mux/3
  Kmax+1/1(X(k)) -> Mux/4
  Kmax+2/1(X(k)) -> Mux/5
  Mux/1 -> DFT/1

== system IEEE5BusSystemModel_opt_UFLS/Subsystem4/PMU_e-IpDFT_P-class/Ia_est/Synchrophasor estimation ==
  DFT : Inport
  dT [s] : Inport  Port=2
  dF [Hz] : Inport  Port=3
  Amplitude - 1 : Subsystem
  Amplitude - 2 : Subsystem
  Complex to Magnitude-Angle1 : ComplexToMagnitudeAngle
  Complex to Magnitude-Angle2 : ComplexToMagnitudeAngle
  Demux1 : Demux  Outputs=5
  Frequency - 2 : Subsystem
  Hanning(Kmax) : Subsystem
  Hanning(Kmax+1) : Subsystem
  Hanning(Kmax-1) : Subsystem
  Phase - 2 : Subsystem
  Terminator : Terminator
  Terminator1 : Terminator
  "delta - 1 " : Subsystem
  delta - 2 : Subsystem
  epsilon : Subsystem
  spectral leakage compensation : Subsystem
  Frequency : Outport  VectorParamsAs1DForOutWhenUnconnected=off
  Amplitude : Outport  Port=2  VectorParamsAs1DForOutWhenUnconnected=off
  Phase : Outport  Port=3  VectorParamsAs1DForOutWhenUnconnected=off
  wires:
  dF [Hz]/1 -> Frequency - 2/2(dF [Hz])
  Hanning(Kmax-1)/1(Hanning out) -> epsilon/1(X (k max -1)), Complex to Magnitude-Angle1/1
  Amplitude - 1/1(amplitude) -> spectral leakage compensation/1(Amplitude)
  dT [s]/1 -> Phase - 2/4(dT [s])
  Complex to Magnitude-Angle2/1 -> Terminator1/1
  Complex to Magnitude-Angle2/2 -> Phase - 2/1(X k_max phase)
  Complex to Magnitude-Angle1/1 -> Terminator/1
  Complex to Magnitude-Angle1/2 -> spectral leakage compensation/6(ph X(k-1))
  Phase - 2/1(phase) -> Phase/1
  delta - 2/1(delta) -> Amplitude - 2/1(delta), Phase - 2/2(delta), Frequency - 2/1(delta)
  spectral leakage compensation/2(X(k max+epsilon)) -> delta - 2/2(X (k max + epsilon))
  spectral leakage compensation/1(X(k max)) -> Amplitude - 2/2((X k_max)), Complex to Magnitude-Angle2/1, delta - 2/1(X (k max))
  "delta - 1 "/1(delta) -> Amplitude - 1/1(delta), spectral leakage compensation/2(delta)
  epsilon/2(epsilon) -> "delta - 1 "/3(epsilon), delta - 2/3(epsilon), spectral leakage compensation/5(epsilon)
  epsilon/1(X (Kmax + epsilon)) -> spectral leakage compensation/3(X (k max + epsilon)), "delta - 1 "/2(X (k max + epsilon))
  Hanning(Kmax)/1(Hanning out) -> spectral leakage compensation/4(X (k max)), Amplitude - 1/2((X k_max)), "delta - 1 "/1(X (k max))
  Hanning(Kmax+1)/1(Hanning out) -> epsilon/2(X (k max+1))
  Demux1/4 -> Hanning(Kmax)/3(Kmax+1), Hanning(Kmax+1)/2(Kmax+1)
  Demux1/3 -> Hanning(Kmax)/2(Kmax), Hanning(Kmax+1)/1(Kmax), Hanning(Kmax-1)/3(Kmax)
  Demux1/2 -> Hanning(Kmax-1)/2(Kmax-1), Hanning(Kmax)/1(Kmax-1)
  Demux1/1 -> Hanning(Kmax-1)/1(Kmax-2)
  Demux1/5 -> Hanning(Kmax+1)/3(Kmax+2)
  Amplitude - 2/1(amplitude) -> Amplitude/1
  Frequency - 2/1(frequency) -> Frequency/1, Phase - 2/3(freq)
  DFT/1 -> Demux1/1

== system IEEE5BusSystemModel_opt_UFLS/Subsystem4/PMU_e-IpDFT_P-class/Ia_est/mSDFT ==
  signal : Inport
  Hit : Inport  Port=2
  Delay_M : Delay  DelayLength=M  SampleTime=Ts_p
  Kmax : Subsystem
  Kmax+1 : Subsystem
  Kmax+2 : Subsystem
  Kmax-1 : Subsystem
  Kmax-2 : Subsystem
  Mux : Mux  Inputs=5
  DFT : Outport  VectorParamsAs1DForOutWhenUnconnected=off
  wires:
  Hit/1 -> Kmax+2/3(trigger), Kmax+1/3(trigger), Kmax/3(trigger), Kmax-1/3(trigger), Kmax-2/3(trigger)
  Delay_M/1 -> Kmax-2/2(x(n-M)), Kmax-1/2(x(n-M)), Kmax+2/2(x(n-M)), Kmax+1/2(x(n-M)), Kmax/2(x(n-M))
  signal/1 -> Delay_M/1, Kmax/1(x(n)), Kmax+1/1(x(n)), Kmax+2/1(x(n)), Kmax-1/1(x(n)), Kmax-2/1(x(n))
  Kmax-2/1(X(k)) -> Mux/1
  Kmax-1/1(X(k)) -> Mux/2
  Kmax/1(X(k)) -> Mux/3
  Kmax+1/1(X(k)) -> Mux/4
  Kmax+2/1(X(k)) -> Mux/5
  Mux/1 -> DFT/1

== system IEEE5BusSystemModel_opt_UFLS/Subsystem4/PMU_e-IpDFT_P-class1/Ia_est/Synchrophasor estimation ==
  DFT : Inport
  dT [s] : Inport  Port=2
  dF [Hz] : Inport  Port=3
  Amplitude - 1 : Subsystem
  Amplitude - 2 : Subsystem
  Complex to Magnitude-Angle1 : ComplexToMagnitudeAngle
  Complex to Magnitude-Angle2 : ComplexToMagnitudeAngle
  Demux1 : Demux  Outputs=5
  Frequency - 2 : Subsystem
  Hanning(Kmax) : Subsystem
  Hanning(Kmax+1) : Subsystem
  Hanning(Kmax-1) : Subsystem
  Phase - 2 : Subsystem
  Terminator : Terminator
  Terminator1 : Terminator
  "delta - 1 " : Subsystem
  delta - 2 : Subsystem
  epsilon : Subsystem
  spectral leakage compensation : Subsystem
  Frequency : Outport  VectorParamsAs1DForOutWhenUnconnected=off
  Amplitude : Outport  Port=2  VectorParamsAs1DForOutWhenUnconnected=off
  Phase : Outport  Port=3  VectorParamsAs1DForOutWhenUnconnected=off
  wires:
  DFT/1 -> Demux1/1
  Frequency - 2/1(frequency) -> Phase - 2/3(freq), Frequency/1
  Amplitude - 2/1(amplitude) -> Amplitude/1
  Demux1/5 -> Hanning(Kmax+1)/3(Kmax+2)
  Demux1/1 -> Hanning(Kmax-1)/1(Kmax-2)
  Demux1/2 -> Hanning(Kmax)/1(Kmax-1), Hanning(Kmax-1)/2(Kmax-1)
  Demux1/3 -> Hanning(Kmax-1)/3(Kmax), Hanning(Kmax+1)/1(Kmax), Hanning(Kmax)/2(Kmax)
  Demux1/4 -> Hanning(Kmax+1)/2(Kmax+1), Hanning(Kmax)/3(Kmax+1)
  Hanning(Kmax+1)/1(Hanning out) -> epsilon/2(X (k max+1))
  Hanning(Kmax)/1(Hanning out) -> "delta - 1 "/1(X (k max)), Amplitude - 1/2((X k_max)), spectral leakage compensation/4(X (k max))
  epsilon/1(X (Kmax + epsilon)) -> "delta - 1 "/2(X (k max + epsilon)), spectral leakage compensation/3(X (k max + epsilon))
  epsilon/2(epsilon) -> spectral leakage compensation/5(epsilon), delta - 2/3(epsilon), "delta - 1 "/3(epsilon)
  "delta - 1 "/1(delta) -> spectral leakage compensation/2(delta), Amplitude - 1/1(delta)
  spectral leakage compensation/1(X(k max)) -> delta - 2/1(X (k max)), Complex to Magnitude-Angle2/1, Amplitude - 2/2((X k_max))
  spectral leakage compensation/2(X(k max+epsilon)) -> delta - 2/2(X (k max + epsilon))
  delta - 2/1(delta) -> Frequency - 2/1(delta), Phase - 2/2(delta), Amplitude - 2/1(delta)
  Phase - 2/1(phase) -> Phase/1
  Complex to Magnitude-Angle1/2 -> spectral leakage compensation/6(ph X(k-1))
  Complex to Magnitude-Angle1/1 -> Terminator/1
  Complex to Magnitude-Angle2/2 -> Phase - 2/1(X k_max phase)
  Complex to Magnitude-Angle2/1 -> Terminator1/1
  dT [s]/1 -> Phase - 2/4(dT [s])
  Amplitude - 1/1(amplitude) -> spectral leakage compensation/1(Amplitude)
  Hanning(Kmax-1)/1(Hanning out) -> Complex to Magnitude-Angle1/1, epsilon/1(X (k max -1))
  dF [Hz]/1 -> Frequency - 2/2(dF [Hz])

== system IEEE5BusSystemModel_opt_UFLS/Subsystem4/PMU_e-IpDFT_P-class1/Ia_est/mSDFT ==
  signal : Inport
  Hit : Inport  Port=2
  Delay_M : Delay  DelayLength=M  SampleTime=Ts_p
  Kmax : Subsystem
  Kmax+1 : Subsystem
  Kmax+2 : Subsystem
  Kmax-1 : Subsystem
  Kmax-2 : Subsystem
  Mux : Mux  Inputs=5
  DFT : Outport  VectorParamsAs1DForOutWhenUnconnected=off
  wires:
  Mux/1 -> DFT/1
  Kmax+2/1(X(k)) -> Mux/5
  Kmax+1/1(X(k)) -> Mux/4
  Kmax/1(X(k)) -> Mux/3
  Kmax-1/1(X(k)) -> Mux/2
  Kmax-2/1(X(k)) -> Mux/1
  signal/1 -> Kmax-2/1(x(n)), Kmax-1/1(x(n)), Kmax+2/1(x(n)), Kmax+1/1(x(n)), Kmax/1(x(n)), Delay_M/1
  Delay_M/1 -> Kmax/2(x(n-M)), Kmax+1/2(x(n-M)), Kmax+2/2(x(n-M)), Kmax-1/2(x(n-M)), Kmax-2/2(x(n-M))
  Hit/1 -> Kmax-2/3(trigger), Kmax-1/3(trigger), Kmax/3(trigger), Kmax+1/3(trigger), Kmax+2/3(trigger)

== system IEEE5BusSystemModel_opt_UFLS/Subsystem5/PMU_e-IpDFT_P-class/Ia_est/Synchrophasor estimation ==
  DFT : Inport
  dT [s] : Inport  Port=2
  dF [Hz] : Inport  Port=3
  Amplitude - 1 : Subsystem
  Amplitude - 2 : Subsystem
  Complex to Magnitude-Angle1 : ComplexToMagnitudeAngle
  Complex to Magnitude-Angle2 : ComplexToMagnitudeAngle
  Demux1 : Demux  Outputs=5
  Frequency - 2 : Subsystem
  Hanning(Kmax) : Subsystem
  Hanning(Kmax+1) : Subsystem
  Hanning(Kmax-1) : Subsystem
  Phase - 2 : Subsystem
  Terminator : Terminator
  Terminator1 : Terminator
  "delta - 1 " : Subsystem
  delta - 2 : Subsystem
  epsilon : Subsystem
  spectral leakage compensation : Subsystem
  Frequency : Outport  VectorParamsAs1DForOutWhenUnconnected=off
  Amplitude : Outport  Port=2  VectorParamsAs1DForOutWhenUnconnected=off
  Phase : Outport  Port=3  VectorParamsAs1DForOutWhenUnconnected=off
  wires:
  dF [Hz]/1 -> Frequency - 2/2(dF [Hz])
  Hanning(Kmax-1)/1(Hanning out) -> epsilon/1(X (k max -1)), Complex to Magnitude-Angle1/1
  Amplitude - 1/1(amplitude) -> spectral leakage compensation/1(Amplitude)
  dT [s]/1 -> Phase - 2/4(dT [s])
  Complex to Magnitude-Angle2/1 -> Terminator1/1
  Complex to Magnitude-Angle2/2 -> Phase - 2/1(X k_max phase)
  Complex to Magnitude-Angle1/1 -> Terminator/1
  Complex to Magnitude-Angle1/2 -> spectral leakage compensation/6(ph X(k-1))
  Phase - 2/1(phase) -> Phase/1
  delta - 2/1(delta) -> Amplitude - 2/1(delta), Phase - 2/2(delta), Frequency - 2/1(delta)
  spectral leakage compensation/2(X(k max+epsilon)) -> delta - 2/2(X (k max + epsilon))
  spectral leakage compensation/1(X(k max)) -> Amplitude - 2/2((X k_max)), Complex to Magnitude-Angle2/1, delta - 2/1(X (k max))
  "delta - 1 "/1(delta) -> Amplitude - 1/1(delta), spectral leakage compensation/2(delta)
  epsilon/2(epsilon) -> "delta - 1 "/3(epsilon), delta - 2/3(epsilon), spectral leakage compensation/5(epsilon)
  epsilon/1(X (Kmax + epsilon)) -> spectral leakage compensation/3(X (k max + epsilon)), "delta - 1 "/2(X (k max + epsilon))
  Hanning(Kmax)/1(Hanning out) -> spectral leakage compensation/4(X (k max)), Amplitude - 1/2((X k_max)), "delta - 1 "/1(X (k max))
  Hanning(Kmax+1)/1(Hanning out) -> epsilon/2(X (k max+1))
  Demux1/4 -> Hanning(Kmax)/3(Kmax+1), Hanning(Kmax+1)/2(Kmax+1)
  Demux1/3 -> Hanning(Kmax)/2(Kmax), Hanning(Kmax+1)/1(Kmax), Hanning(Kmax-1)/3(Kmax)
  Demux1/2 -> Hanning(Kmax-1)/2(Kmax-1), Hanning(Kmax)/1(Kmax-1)
  Demux1/1 -> Hanning(Kmax-1)/1(Kmax-2)
  Demux1/5 -> Hanning(Kmax+1)/3(Kmax+2)
  Amplitude - 2/1(amplitude) -> Amplitude/1
  Frequency - 2/1(frequency) -> Frequency/1, Phase - 2/3(freq)
  DFT/1 -> Demux1/1

== system IEEE5BusSystemModel_opt_UFLS/Subsystem5/PMU_e-IpDFT_P-class/Ia_est/mSDFT ==
  signal : Inport
  Hit : Inport  Port=2
  Delay_M : Delay  DelayLength=M  SampleTime=Ts_p
  Kmax : Subsystem
  Kmax+1 : Subsystem
  Kmax+2 : Subsystem
  Kmax-1 : Subsystem
  Kmax-2 : Subsystem
  Mux : Mux  Inputs=5
  DFT : Outport  VectorParamsAs1DForOutWhenUnconnected=off
  wires:
  Hit/1 -> Kmax+2/3(trigger), Kmax+1/3(trigger), Kmax/3(trigger), Kmax-1/3(trigger), Kmax-2/3(trigger)
  Delay_M/1 -> Kmax-2/2(x(n-M)), Kmax-1/2(x(n-M)), Kmax+2/2(x(n-M)), Kmax+1/2(x(n-M)), Kmax/2(x(n-M))
  signal/1 -> Delay_M/1, Kmax/1(x(n)), Kmax+1/1(x(n)), Kmax+2/1(x(n)), Kmax-1/1(x(n)), Kmax-2/1(x(n))
  Kmax-2/1(X(k)) -> Mux/1
  Kmax-1/1(X(k)) -> Mux/2
  Kmax/1(X(k)) -> Mux/3
  Kmax+1/1(X(k)) -> Mux/4
  Kmax+2/1(X(k)) -> Mux/5
  Mux/1 -> DFT/1

== system IEEE5BusSystemModel_opt_UFLS/Subsystem5/PMU_e-IpDFT_P-class1/Ia_est/Synchrophasor estimation ==
  DFT : Inport
  dT [s] : Inport  Port=2
  dF [Hz] : Inport  Port=3
  Amplitude - 1 : Subsystem
  Amplitude - 2 : Subsystem
  Complex to Magnitude-Angle1 : ComplexToMagnitudeAngle
  Complex to Magnitude-Angle2 : ComplexToMagnitudeAngle
  Demux1 : Demux  Outputs=5
  Frequency - 2 : Subsystem
  Hanning(Kmax) : Subsystem
  Hanning(Kmax+1) : Subsystem
  Hanning(Kmax-1) : Subsystem
  Phase - 2 : Subsystem
  Terminator : Terminator
  Terminator1 : Terminator
  "delta - 1 " : Subsystem
  delta - 2 : Subsystem
  epsilon : Subsystem
  spectral leakage compensation : Subsystem
  Frequency : Outport  VectorParamsAs1DForOutWhenUnconnected=off
  Amplitude : Outport  Port=2  VectorParamsAs1DForOutWhenUnconnected=off
  Phase : Outport  Port=3  VectorParamsAs1DForOutWhenUnconnected=off
  wires:
  DFT/1 -> Demux1/1
  Frequency - 2/1(frequency) -> Phase - 2/3(freq), Frequency/1
  Amplitude - 2/1(amplitude) -> Amplitude/1
  Demux1/5 -> Hanning(Kmax+1)/3(Kmax+2)
  Demux1/1 -> Hanning(Kmax-1)/1(Kmax-2)
  Demux1/2 -> Hanning(Kmax)/1(Kmax-1), Hanning(Kmax-1)/2(Kmax-1)
  Demux1/3 -> Hanning(Kmax-1)/3(Kmax), Hanning(Kmax+1)/1(Kmax), Hanning(Kmax)/2(Kmax)
  Demux1/4 -> Hanning(Kmax+1)/2(Kmax+1), Hanning(Kmax)/3(Kmax+1)
  Hanning(Kmax+1)/1(Hanning out) -> epsilon/2(X (k max+1))
  Hanning(Kmax)/1(Hanning out) -> "delta - 1 "/1(X (k max)), Amplitude - 1/2((X k_max)), spectral leakage compensation/4(X (k max))
  epsilon/1(X (Kmax + epsilon)) -> "delta - 1 "/2(X (k max + epsilon)), spectral leakage compensation/3(X (k max + epsilon))
  epsilon/2(epsilon) -> spectral leakage compensation/5(epsilon), delta - 2/3(epsilon), "delta - 1 "/3(epsilon)
  "delta - 1 "/1(delta) -> spectral leakage compensation/2(delta), Amplitude - 1/1(delta)
  spectral leakage compensation/1(X(k max)) -> delta - 2/1(X (k max)), Complex to Magnitude-Angle2/1, Amplitude - 2/2((X k_max))
  spectral leakage compensation/2(X(k max+epsilon)) -> delta - 2/2(X (k max + epsilon))
  delta - 2/1(delta) -> Frequency - 2/1(delta), Phase - 2/2(delta), Amplitude - 2/1(delta)
  Phase - 2/1(phase) -> Phase/1
  Complex to Magnitude-Angle1/2 -> spectral leakage compensation/6(ph X(k-1))
  Complex to Magnitude-Angle1/1 -> Terminator/1
  Complex to Magnitude-Angle2/2 -> Phase - 2/1(X k_max phase)
  Complex to Magnitude-Angle2/1 -> Terminator1/1
  dT [s]/1 -> Phase - 2/4(dT [s])
  Amplitude - 1/1(amplitude) -> spectral leakage compensation/1(Amplitude)
  Hanning(Kmax-1)/1(Hanning out) -> Complex to Magnitude-Angle1/1, epsilon/1(X (k max -1))
  dF [Hz]/1 -> Frequency - 2/2(dF [Hz])

== system IEEE5BusSystemModel_opt_UFLS/Subsystem5/PMU_e-IpDFT_P-class1/Ia_est/mSDFT ==
  signal : Inport
  Hit : Inport  Port=2
  Delay_M : Delay  DelayLength=M  SampleTime=Ts_p
  Kmax : Subsystem
  Kmax+1 : Subsystem
  Kmax+2 : Subsystem
  Kmax-1 : Subsystem
  Kmax-2 : Subsystem
  Mux : Mux  Inputs=5
  DFT : Outport  VectorParamsAs1DForOutWhenUnconnected=off
  wires:
  Mux/1 -> DFT/1
  Kmax+2/1(X(k)) -> Mux/5
  Kmax+1/1(X(k)) -> Mux/4
  Kmax/1(X(k)) -> Mux/3
  Kmax-1/1(X(k)) -> Mux/2
  Kmax-2/1(X(k)) -> Mux/1
  signal/1 -> Kmax-2/1(x(n)), Kmax-1/1(x(n)), Kmax+2/1(x(n)), Kmax+1/1(x(n)), Kmax/1(x(n)), Delay_M/1
  Delay_M/1 -> Kmax/2(x(n-M)), Kmax+1/2(x(n-M)), Kmax+2/2(x(n-M)), Kmax-1/2(x(n-M)), Kmax-2/2(x(n-M))
  Hit/1 -> Kmax-2/3(trigger), Kmax-1/3(trigger), Kmax/3(trigger), Kmax+1/3(trigger), Kmax+2/3(trigger)

== system IEEE5BusSystemModel_opt_UFLS/Subsystem1/PMU_e-IpDFT_P-class/Ia_est/Synchrophasor estimation/Amplitude - 1 ==
  delta : Inport
  (X k_max) : Inport  Port=2
  Abs1 : Abs
  Abs2 : Abs
  Abs3 : Abs
  Constant : Constant  SampleTime=Ts_p
  Constant2 : Constant  SampleTime=Ts_p
  Fcn1 : Fcn  Expr=(pi*u)/sin(pi*u)
  Gain : Gain  Gain=-1
  Product : Product  RndMeth=Zero
  Product2 : Product  Inputs=3  RndMeth=Zero
  Sum : Sum  Inputs=|++
  Switch1 : Switch  Criteria=u2 ~= 0
  amplitude : Outport  VectorParamsAs1DForOutWhenUnconnected=off
  wires:
  Abs2/1 -> Product2/1
  Product/1 -> Gain/1
  Sum/1 -> Product2/3
  Constant/1 -> Sum/2
  Abs1/1 -> Product2/2
  Switch1/1 -> Abs2/1
  Constant2/1 -> Switch1/3
  Abs3/1 -> Switch1/2
  Fcn1/1 -> Switch1/1
  (X k_max)/1 -> Abs1/1
  Product2/1 -> amplitude/1
  delta/1 -> Product/1, Product/2, Abs3/1, Fcn1/1
  Gain/1 -> Sum/1

== system IEEE5BusSystemModel_opt_UFLS/Subsystem1/PMU_e-IpDFT_P-class/Ia_est/Synchrophasor estimation/Amplitude - 2 ==
  delta : Inport
  (X k_max) : Inport  Port=2
  Abs1 : Abs
  Abs2 : Abs
  Abs3 : Abs
  Constant : Constant  SampleTime=Inf
  Constant2 : Constant  SampleTime=Ts_p
  Fcn1 : Fcn  Expr=(pi*u)/sin(pi*u)
  Gain : Gain  Gain=-1
  Gain1 : Gain  Gain=sqrt(2)
  Product : Product  RndMeth=Zero
  Product2 : Product  Inputs=3  RndMeth=Zero
  Sum : Sum  Inputs=|++
  Switch1 : Switch  Criteria=u2 ~= 0
  amplitude : Outport  VectorParamsAs1DForOutWhenUnconnected=off
  wires:
  Abs2/1 -> Product2/1
  Product/1 -> Gain/1
  Sum/1 -> Product2/3
  Constant/1 -> Sum/2
  Abs1/1 -> Product2/2
  Switch1/1 -> Abs2/1
  Constant2/1 -> Switch1/3
  Abs3/1 -> Switch1/2
  Fcn1/1 -> Switch1/1
  (X k_max)/1 -> Abs1/1
  Product2/1 -> Gain1/1
  delta/1 -> Product/1, Product/2, Abs3/1, Fcn1/1
  Gain/1 -> Sum/1
  Gain1/1 -> amplitude/1

== system IEEE5BusSystemModel_opt_UFLS/Subsystem1/PMU_e-IpDFT_P-class/Ia_est/Synchrophasor estimation/Frequency - 2 ==
  delta : Inport
  dF [Hz] : Inport  Port=2
  Add : Sum
  Constant1 : Constant  Value=kmax  SampleTime=Ts_p
  Product : Product  RndMeth=Zero
  frequency : Outport  VectorParamsAs1DForOutWhenUnconnected=off
  wires:
  Add/1 -> Product/2
  Constant1/1 -> Add/1
  delta/1 -> Add/2
  Product/1 -> frequency/1
  dF [Hz]/1 -> Product/1

== system IEEE5BusSystemModel_opt_UFLS/Subsystem1/PMU_e-IpDFT_P-class/Ia_est/Synchrophasor estimation/Hanning(Kmax) ==
  Kmax-1 : Inport
  Kmax : Inport  Port=2
  Kmax+1 : Inport  Port=3
  Add1 : Sum  Inputs=+++
  Constant3 : Constant  Value=-0.25  SampleTime=Ts_p
  Constant4 : Constant  Value=0.5  SampleTime=Ts_p
  Constant5 : Constant  Value=-0.25  SampleTime=Ts_p
  Product3 : Product  RndMeth=Zero
  Product4 : Product  RndMeth=Zero
  Product5 : Product  RndMeth=Zero
  Hanning out : Outport  VectorParamsAs1DForOutWhenUnconnected=off
  wires:
  Add1/1 -> Hanning out/1
  Kmax+1/1 -> Product5/1
  Kmax/1 -> Product4/1
  Kmax-1/1 -> Product3/1
  Product5/1 -> Add1/3
  Product4/1 -> Add1/2
  Product3/1 -> Add1/1
  Constant4/1 -> Product4/2
  Constant5/1 -> Product5/2
  Constant3/1 -> Product3/2

== system IEEE5BusSystemModel_opt_UFLS/Subsystem1/PMU_e-IpDFT_P-class/Ia_est/Synchrophasor estimation/Hanning(Kmax+1) ==
  Kmax : Inport
  Kmax+1 : Inport  Port=2
  Kmax+2 : Inport  Port=3
  Add2 : Sum  Inputs=+++
  Constant6 : Constant  Value=-0.25  SampleTime=Ts_p
  Constant7 : Constant  Value=0.5  SampleTime=Ts_p
  Constant8 : Constant  Value=-0.25  SampleTime=Ts_p
  Product6 : Product  RndMeth=Zero
  Product7 : Product  RndMeth=Zero
  Product8 : Product  RndMeth=Zero
  Hanning out : Outport  VectorParamsAs1DForOutWhenUnconnected=off
  wires:
  Kmax+2/1 -> Product8/1
  Add2/1 -> Hanning out/1
  Kmax+1/1 -> Product7/1
  Kmax/1 -> Product6/1
  Product8/1 -> Add2/3
  Product7/1 -> Add2/2
  Product6/1 -> Add2/1
  Constant7/1 -> Product7/2
  Constant8/1 -> Product8/2
  Constant6/1 -> Product6/2

== system IEEE5BusSystemModel_opt_UFLS/Subsystem1/PMU_e-IpDFT_P-class/Ia_est/Synchrophasor estimation/Hanning(Kmax-1) ==
  Kmax-2 : Inport
  Kmax-1 : Inport  Port=2
  Kmax : Inport  Port=3
  Add : Sum  Inputs=+++
  Constant : Constant  Value=-0.25  SampleTime=Ts_p
  Constant1 : Constant  Value=0.5  SampleTime=Ts_p
  Constant2 : Constant  Value=-0.25  SampleTime=Ts_p
  Product : Product  RndMeth=Zero
  Product1 : Product  RndMeth=Zero
  Product2 : Product  RndMeth=Zero
  Hanning out : Outport  VectorParamsAs1DForOutWhenUnconnected=off
  wires:
  Add/1 -> Hanning out/1
  Kmax-2/1 -> Product/1
  Kmax/1 -> Product2/1
  Kmax-1/1 -> Product1/1
  Product2/1 -> Add/3
  Product1/1 -> Add/2
  Product/1 -> Add/1
  Constant1/1 -> Product1/2
  Constant2/1 -> Product2/2
  Constant/1 -> Product/2

== system IEEE5BusSystemModel_opt_UFLS/Subsystem1/PMU_e-IpDFT_P-class/Ia_est/Synchrophasor estimation/Phase - 2 ==
  X k_max phase : Inport
  delta : Inport  Port=2
  freq : Inport  Port=3
  dT [s] : Inport  Port=4
  Add1 : Sum  Inputs=+-
  Add3 : Sum  Inputs=+++
  Constant3 : Constant  Value=pi  SampleTime=Ts_p
  Constant5 : Constant  Value=2*pi  SampleTime=Ts_p
  Gain : Gain  Gain=2*pi*T/2
  Product : Product  RndMeth=Zero
  Product1 : Product  Inputs=3  RndMeth=Zero
  WrapToPi : Subsystem
  phase : Outport  VectorParamsAs1DForOutWhenUnconnected=off
  wires:
  Product1/1 -> Add3/3
  Gain/1 -> Add3/2
  Add3/1 -> WrapToPi/1(angle in)
  Add1/1 -> Add3/1
  WrapToPi/1(angle out) -> phase/1
  freq/1 -> Gain/1, Product1/1
  dT [s]/1 -> Product1/3
  Constant5/1 -> Product1/2
  Product/1 -> Add1/2
  delta/1 -> Product/1
  X k_max phase/1 -> Add1/1
  Constant3/1 -> Product/2

== system IEEE5BusSystemModel_opt_UFLS/Subsystem1/PMU_e-IpDFT_P-class/Ia_est/Synchrophasor estimation/delta - 1  ==
  X (k max) : Inport
  X (k max + epsilon) : Inport  Port=2
  epsilon : Inport  Port=3
  Abs2 : Abs
  Abs4 : Abs
  Divide : Product  Inputs=*/
  Gain : Gain  Gain=2
  Product : Product  RndMeth=Zero
  Subtract : Sum  Inputs=+-
  Subtract1 : Sum
  delta : Outport  VectorParamsAs1DForOutWhenUnconnected=off
  wires:
  epsilon/1 -> Product/1
  Product/1 -> delta/1
  Divide/1 -> Product/2
  Subtract1/1 -> Divide/2
  Subtract/1 -> Divide/1
  X (k max + epsilon)/1 -> Abs2/1
  X (k max)/1 -> Abs4/1
  Gain/1 -> Subtract/1
  Abs4/1 -> Subtract1/2, Subtract/2
  Abs2/1 -> Subtract1/1, Gain/1
